simulink model "ModelodeRisco"  (R2024a)
settings: Solver=VariableStepAuto  StartTime=0.0  StopTime=10.0  RelTol=1e-3
values from neighbouring files (symbols this model uses):
  hight_max = 5    [atv.m]
  hight_min = 0    [atv.m]
  i_hight = std(hight)    [atv.m]
  i_temp = std(temp)    [atv.m]
  i_turb = std(turb)    [atv.m]
  m_hight = mean(hight)    [atv.m]
  m_temp = mean(temp)    [atv.m]
  m_turb = mean(turb)    [atv.m]
  temp_max = 30    [atv.m]
  temp_min = 15    [atv.m]
  turb_max = 5    [atv.m]
  turb_min = 0    [atv.m]

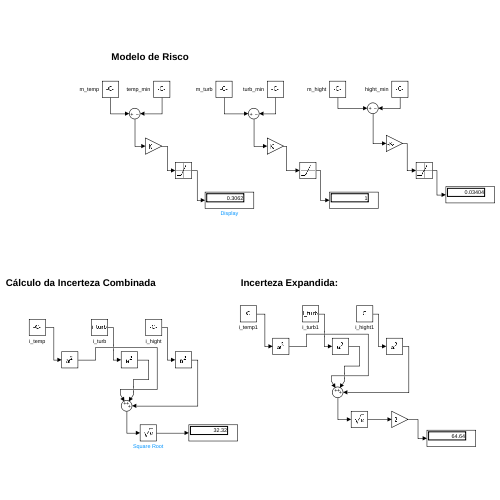
[thumbnail: Simulink's stored preview of the top-level diagram]
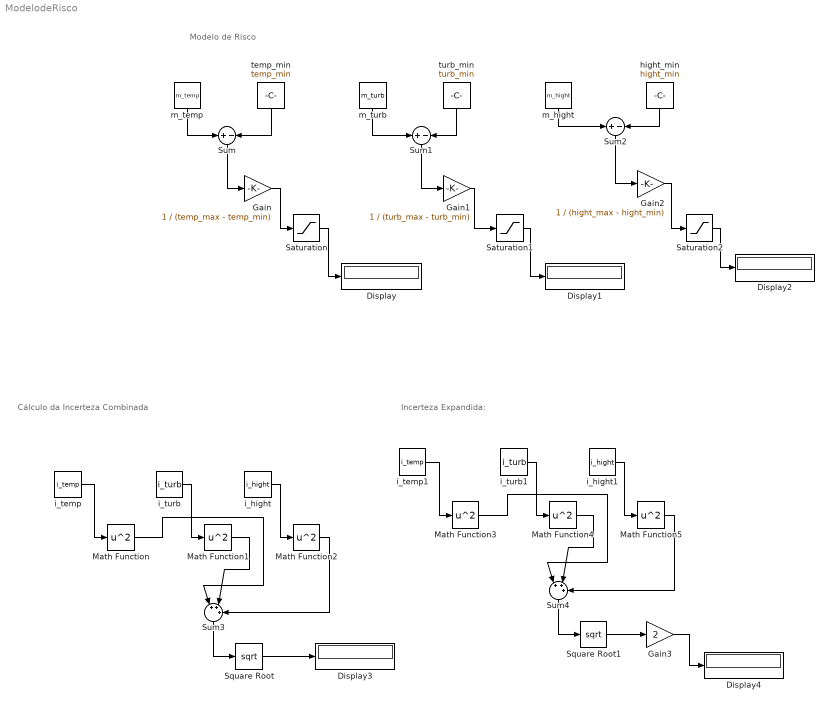
== system ModelodeRisco ==
  note: Modelo de Risco
  note: Incerteza Expandida:
  note: Cálculo da Incerteza Combinada
  Display{,1..4} (5 alike) : Display
  Gain : Gain  Gain=1 / (temp_max - temp_min)
  Gain1 : Gain  Gain=1 / (turb_max - turb_min)
  Gain2 : Gain  Gain=1 / (hight_max - hight_min)
  Gain3 : Gain  Gain=2
  Math Function{,1..5} (6 alike) : Math  Operator=square
  Saturation : Saturate  UpperLimit=1  LowerLimit=0
  Saturation1 : Saturate  UpperLimit=1  LowerLimit=0
  Saturation2 : Saturate  UpperLimit=1  LowerLimit=0
  Square Root : Sqrt
  Square Root1 : Sqrt
  Sum : Sum  Inputs=+-
  Sum1 : Sum  Inputs=+-
  Sum2 : Sum  Inputs=+-
  Sum3 : Sum  Inputs=|+++
  Sum4 : Sum  Inputs=|+++
  hight_min : Constant  Value=hight_min
  i_hight : Constant  Value=i_hight
  i_hight1 : Constant  Value=i_hight
  i_temp : Constant  Value=i_temp
  i_temp1 : Constant  Value=i_temp
  i_turb : Constant  Value=i_turb
  i_turb1 : Constant  Value=i_turb
  m_hight : Constant  Value=m_hight
  m_temp : Constant  Value=m_temp
  m_turb : Constant  Value=m_turb
  temp_min : Constant  Value=temp_min
  turb_min : Constant  Value=turb_min
  wires:
  m_temp/1 -> Sum/1
  temp_min/1 -> Sum/2
  m_turb/1 -> Sum1/1
  turb_min/1 -> Sum1/2
  m_hight/1 -> Sum2/1
  hight_min/1 -> Sum2/2
  Sum/1 -> Gain/1
  Sum1/1 -> Gain1/1
  Sum2/1 -> Gain2/1
  Gain/1 -> Saturation/1
  Gain1/1 -> Saturation1/1
  Gain2/1 -> Saturation2/1
  Saturation/1 -> Display/1
  Saturation1/1 -> Display1/1
  Saturation2/1 -> Display2/1
  i_temp/1 -> Math Function/1
  Math Function/1 -> Sum3/1
  Math Function1/1 -> Sum3/2
  Math Function2/1 -> Sum3/3
  i_turb/1 -> Math Function1/1
  i_hight/1 -> Math Function2/1
  Sum3/1 -> Square Root/1
  Square Root/1 -> Display3/1
  Sum4/1 -> Square Root1/1
  i_turb1/1 -> Math Function4/1
  Math Function3/1 -> Sum4/1
  i_temp1/1 -> Math Function3/1
  Math Function5/1 -> Sum4/3
  i_hight1/1 -> Math Function5/1
  Math Function4/1 -> Sum4/2
  Square Root1/1 -> Gain3/1
  Gain3/1 -> Display4/1
